simulink model "Model"  (R2023a)
settings: Solver=FixedStepAuto  StartTime=0.0  StopTime=4  FixedStep=0.0001  RelTol=1e-3
values from neighbouring files (symbols this model uses):
  J2 = 1.26e-3    (= 0.00126)    [system_init.m]
libraries: dspfdesign x4
settings Model: SimulationMode=accelerator  Creator=04  LastModifiedBy=23688
settings SolverCC: AlgebraicLoopSolver=TrustRegion
settings DataIOCC: ReturnWorkspaceOutputs=off
settings DebuggingCC: UnconnectedInputMsg=warning  UnconnectedOutputMsg=warning  UnconnectedLineMsg=warning
settings ModelReferenceCC: EnableRefExpFcnMdlSchedulingChecks=on
settings RTWCC: DLArmComputeVersion=19.05

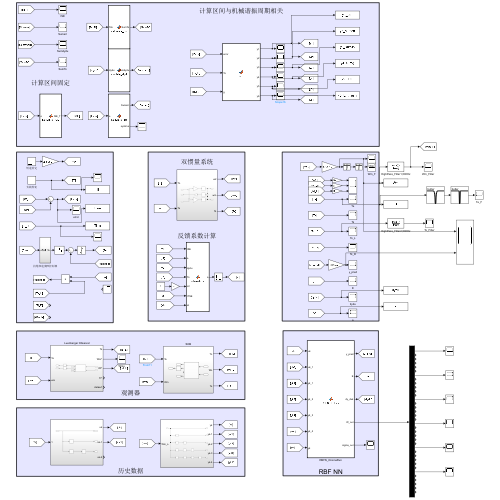
[thumbnail: Simulink's stored preview of the top-level diagram]
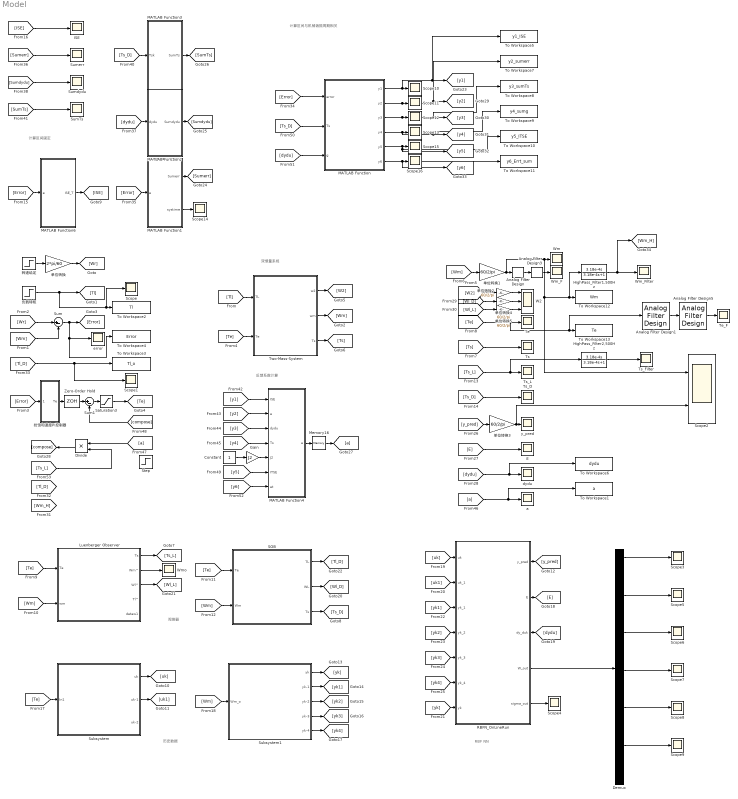
== system Model ==
  note: 观测器
  note: 历史数据
  note: 计算区间固定
  note: 计算区间与机械谐振周期相关
  note: 双惯量系统
  note: 反馈系数计算
  note: RBF NN
  " Luenberger Observer" : Subsystem
  Analog Filter Design : dspfdesign/Analog Filter Design  method=Butterworth  filttype=Bandstop  N=12  Wlo=700*2*pi  Whi=1300*2*pi  Rp=2  Rs=40
  Analog Filter Design1 : dspfdesign/Analog Filter Design  method=Butterworth  filttype=Bandstop  N=2  Wlo=700*2*pi  Whi=1300*2*pi  Rp=2  Rs=40
  Analog Filter Design3 : dspfdesign/Analog Filter Design  method=Butterworth  filttype=Bandstop  N=12  Wlo=900*2*pi  Whi=1100*2*pi  Rp=2  Rs=40
  Analog Filter Design5 : dspfdesign/Analog Filter Design  method=Butterworth  filttype=Bandstop  N=2  Wlo=950*2*pi  Whi=1050*2*pi  Rp=2  Rs=40
  Constant : Constant
  Demux : Demux  Outputs=36
  Divide : Product  Inputs=**
  E : Scope
  Gain : Gain  Gain=J2
  HighPass_Filter1,500Hz : TransferFcn  Numerator=[3.18e-4 0]  Denominator=[3.18e-4 1]
  HighPass_Filter2,500Hz : TransferFcn  Numerator=[3.18e-4 0]  Denominator=[3.18e-4 1]
  ISE : Scope
  MATLAB Function : MATLAB Function  TreatAsAtomicUnit=on
  MATLAB Function1 : MATLAB Function  TreatAsAtomicUnit=on
  MATLAB Function2 : MATLAB Function  TreatAsAtomicUnit=on
  MATLAB Function3 : MATLAB Function  TreatAsAtomicUnit=on
  MATLAB Function4 : MATLAB Function  TreatAsAtomicUnit=on
  MATLAB Function6 : MATLAB Function  TreatAsAtomicUnit=on
  Memory16 : Memory  InheritSampleTime=on
  RBFN_OnLineRun : MATLAB Function  TreatAsAtomicUnit=on
  SOB : Subsystem
  Saturation3 : Saturate  UpperLimit=2.39*3  LowerLimit=-2.39*3
  Scope{,1,3..16} (16 alike) : Scope
  Scope2 : Scope  NumInputPorts=2
  Step : Step  Time=1.2  After=0  SampleTime=0
  Subsystem : Subsystem
  Subsystem1 : Subsystem
  Sum : Sum  Inputs=|+-
  Sum1 : Sum  Inputs=|+-
  SumTs : Scope
  Sumdydu : Scope
  Sumerr : Scope
  Te : Scope
  Te_F : Scope
  To Workspace1 : ToWorkspace  VariableName=a  SampleTime=-1
  To Workspace10 : ToWorkspace  VariableName=y5_ITSE  SampleTime=-1
  To Workspace11 : ToWorkspace  VariableName=y6_Errt_sum  SampleTime=-1
  To Workspace12 : ToWorkspace  VariableName=Wm  SampleTime=-1
  To Workspace13 : ToWorkspace  VariableName=Te  SampleTime=-1
  To Workspace2 : ToWorkspace  VariableName=Tl  SampleTime=-1
  To Workspace3 : ToWorkspace  VariableName=Tl_o  SampleTime=-1
  To Workspace4 : ToWorkspace  VariableName=Error  SampleTime=-1
  To Workspace5 : ToWorkspace  VariableName=y1_ISE  SampleTime=-1
  To Workspace6 : ToWorkspace  VariableName=dydu  SampleTime=-1
  To Workspace7 : ToWorkspace  VariableName=y2_sumerr  SampleTime=-1
  To Workspace8 : ToWorkspace  VariableName=y3_sumTs  SampleTime=-1
  To Workspace9 : ToWorkspace  VariableName=y4_sumg  SampleTime=-1
  Ts : Scope
  Ts_D : Scope
  Ts_Filter : Scope
  Ts_L : Scope
  Two-Mass-System : Subsystem
  W2 : Scope  NumInputPorts=3
  Wm : Scope
  Wm_F : Scope
  Wm_Filter : Scope
  Wmo : Scope
  Zero-Order Hold : ZeroOrderHold  SampleTime=0.0005
  a : Scope
  dydu : Scope
  error : Scope
  y_pred : Scope
  单位转换 : Gain  Gain=2*pi/60
  单位转换{1..5} (5 alike) : Gain  Gain=60/2/pi
  抗饱和速度PI控制器 : Subsystem
  负载转矩 : Step  Time=0  After=0  SampleTime=0
  转速给定 : Step  Time=0.1  After=1000  SampleTime=0
  wires:
  负载转矩/1 -> Scope/1, To Workspace2/1, [Tl]
  [Tl] -> Two-Mass-System/1(TL)
  Two-Mass-System/2(wm) -> [Wm]
  [Wr] -> Sum/1
  [Wm] -> Sum/2
  Sum/1 -> To Workspace4/1, error/1, [Error]
  [Error] -> 抗饱和速度PI控制器/1(error)
  Two-Mass-System/1(w2) -> [W2]
  Two-Mass-System/3(Ts) -> [Ts]
  [Ts] -> Ts/1
  单位转换/1 -> [Wr]
  [Wm] -> 单位转换1/1
  [Te] -> " Luenberger Observer"/1(Te)
  [Wm] -> " Luenberger Observer"/2(wm)
  [Te] -> SOB/1(Te)
  [Wm] -> SOB/2(Wm)
  " Luenberger Observer"/1(Ts) -> [Ts_L]
  SOB/3(Ts) -> [Ts_D]
  [Ts_L] -> HighPass_Filter2,500Hz/1, Ts_L/1
  [Ts_D] -> Ts_D/1
  [W2] -> 单位转换2/1
  单位转换2/1 -> W2/1
  [Te] -> Subsystem/1(In1)
  Subsystem/1(uk) -> [uk]
  Subsystem/2(uk-1) -> [uk1]
  [Wm] -> Subsystem1/1(Wm_o)
  Subsystem1/1(yk) -> [yk]
  Subsystem1/2(yk-1) -> [yk1]
  Subsystem1/3(yk-2) -> [yk2]
  Subsystem1/4(yk-3) -> [yk3]
  Subsystem1/5(yk-4) -> [yk4]
  [uk] -> RBFN_OnLineRun/1(uk)
  [uk1] -> RBFN_OnLineRun/2(uk_1)
  [yk] -> RBFN_OnLineRun/7(yk)
  [yk1] -> RBFN_OnLineRun/3(yk_1)
  [yk2] -> RBFN_OnLineRun/4(yk_2)
  [yk3] -> RBFN_OnLineRun/5(yk_3)
  [yk4] -> RBFN_OnLineRun/6(yk_4)
  RBFN_OnLineRun/1(y_pred) -> [y_pred]
  RBFN_OnLineRun/2(E) -> [E]
  [E] -> E/1
  [dydu] -> To Workspace6/1, dydu/1
  [y_pred] -> 单位转换3/1
  单位转换3/1 -> Scope2/2, y_pred/1
  SOB/2(WL) -> [Wl_D]
  " Luenberger Observer"/3(Wl^) -> [Wl_L]
  单位转换4/1 -> W2/2
  [Wl_D] -> 单位转换4/1
  单位转换5/1 -> W2/3
  [Wl_L] -> 单位转换5/1
  Analog Filter Design/1 -> Analog Filter Design3/1
  Analog Filter Design3/1 -> Wm_F/1
  单位转换1/1 -> Scope2/1, HighPass_Filter1,500Hz/1, To Workspace12/1, Wm/1, Analog Filter Design/1
  [Error] -> MATLAB Function1/1(e)
  MATLAB Function1/1(Sumerr) -> [Sumerr]
  [ISE] -> ISE/1
  [Sumerr] -> Sumerr/1
  [dydu] -> MATLAB Function2/1(dydu)
  MATLAB Function2/1(Sumdydu) -> [Sumdydu]
  [Sumdydu] -> Sumdydu/1
  [Ts_D] -> MATLAB Function3/1(Tsk)
  MATLAB Function3/1(SumTs) -> [SumTs]
  [SumTs] -> SumTs/1
  [y1] -> MATLAB Function4/1(ISE)
  [y2] -> MATLAB Function4/2(e)
  [y3] -> MATLAB Function4/3(dydu)
  [y4] -> MATLAB Function4/4(Ts)
  [a] -> To Workspace1/1, a/1
  Divide/1 -> [compose]
  [Te] -> Two-Mass-System/2(Te)
  MATLAB Function6/1(ISE_T) -> [ISE]
  [Error] -> MATLAB Function6/1(e)
  Gain/1 -> MATLAB Function4/5(J2)
  Constant/1 -> Gain/1
  SOB/1(TL) -> [Tl_D]
  [Tl_D] -> To Workspace3/1, Scope1/1
  [Te] -> Analog Filter Design1/1, To Workspace13/1, Te/1
  RBFN_OnLineRun/4(W_out) -> Demux/1
  Demux/1 -> Scope3/1
  RBFN_OnLineRun/5(sigma_out) -> Scope4/1
  Demux/7 -> Scope5/1
  Demux/13 -> Scope6/1
  Demux/19 -> Scope7/1
  Demux/25 -> Scope8/1
  Demux/31 -> Scope9/1
  [compose] -> Sum1/2
  抗饱和速度PI控制器/1(Te) -> Zero-Order Hold/1
  Zero-Order Hold/1 -> Sum1/1
  [Error] -> MATLAB Function/1(error)
  MATLAB Function/1(y1) -> Scope10/1, To Workspace5/1, [y1]
  MATLAB Function/2(y2) -> Scope11/1, To Workspace7/1, [y2]
  [Ts_D] -> MATLAB Function/2(Ts)
  MATLAB Function/3(y3) -> To Workspace8/1, [y3], Scope12/1
  [dydu] -> MATLAB Function/3(g)
  MATLAB Function/4(y4) -> To Workspace9/1, [y4], Scope13/1
  MATLAB Function4/1(a) -> Memory16/1
  RBFN_OnLineRun/3(dy_duk) -> [dydu]
  Memory16/1 -> [a]
  MATLAB Function1/2(systime) -> Scope14/1
  MATLAB Function/5(y5) -> [y5], To Workspace10/1, Scope15/1
  [y5] -> MATLAB Function4/6(ITSE)
  MATLAB Function/6(y6) -> [y6], To Workspace11/1, Scope16/1
  [y6] -> MATLAB Function4/7(et)
  Analog Filter Design1/1 -> Analog Filter Design5/1
  Analog Filter Design5/1 -> Te_F/1
  HighPass_Filter2,500Hz/1 -> Ts_Filter/1
  HighPass_Filter1,500Hz/1 -> [Wm_H], Wm_Filter/1
  Sum1/1 -> Saturation3/1
  Saturation3/1 -> [Te]
  " Luenberger Observer"/2(Wm^) -> Wmo/1
  转速给定/1 -> 单位转换/1
  [Ts_L] -> Divide/2
  [a] -> Divide/1

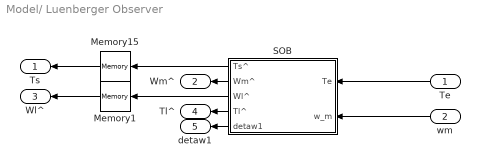
== system Model/ Luenberger Observer ==
  Te : Inport
  wm : Inport  Port=2
  Memory1 : Memory
  Memory15 : Memory
  SOB : Subsystem
  Ts : Outport
  Wm^ : Outport  Port=2
  Wl^ : Outport  Port=3
  Tl^ : Outport  Port=4
  detaw1 : Outport  Port=5
  wires:
  SOB/4(Tl^) -> Tl^/1
  SOB/1(Ts^) -> Memory15/1
  Memory15/1 -> Ts/1
  wm/1 -> SOB/2(w_m)
  SOB/2(Wm^) -> Wm^/1
  Te/1 -> SOB/1(Te)
  SOB/5(detaw1) -> detaw1/1
  Memory1/1 -> Wl^/1
  SOB/3(Wl^) -> Memory1/1

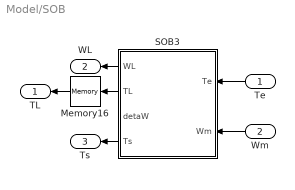
== system Model/SOB ==
  Te : Inport
  Wm : Inport  Port=2
  Memory16 : Memory
  SOB3 : Subsystem
  TL : Outport
  WL : Outport  Port=2
  Ts : Outport  Port=3
  wires:
  SOB3/1(WL) -> WL/1
  SOB3/4(Ts) -> Ts/1
  Wm/1 -> SOB3/2(Wm)
  Te/1 -> SOB3/1(Te)
  SOB3/2(TL) -> Memory16/1
  Memory16/1 -> TL/1

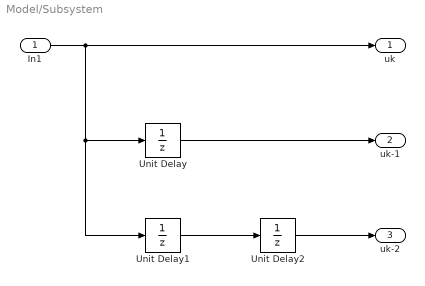
== system Model/Subsystem ==
  In1 : Inport
  Unit Delay : UnitDelay  SampleTime=-1  HasFrameUpgradeWarning=on
  Unit Delay1 : UnitDelay  SampleTime=-1  HasFrameUpgradeWarning=on
  Unit Delay2 : UnitDelay  SampleTime=-1  HasFrameUpgradeWarning=on
  uk : Outport
  uk-1 : Outport  Port=2
  uk-2 : Outport  Port=3
  wires:
  Unit Delay1/1 -> Unit Delay2/1
  Unit Delay/1 -> uk-1/1
  Unit Delay2/1 -> uk-2/1
  In1/1 -> Unit Delay1/1, Unit Delay/1, uk/1

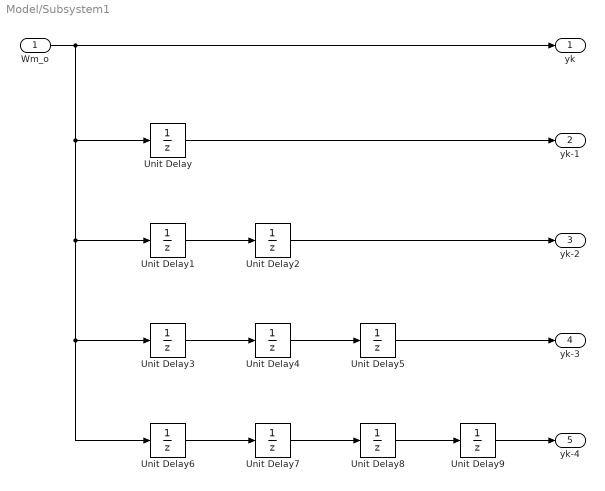
== system Model/Subsystem1 ==
  Wm_o : Inport
  Unit Delay{,1..9} (10 alike) : UnitDelay  SampleTime=-1  HasFrameUpgradeWarning=on
  yk : Outport
  yk-1 : Outport  Port=2
  yk-2 : Outport  Port=3
  yk-3 : Outport  Port=4
  yk-4 : Outport  Port=5
  wires:
  Unit Delay5/1 -> yk-3/1
  Unit Delay4/1 -> Unit Delay5/1
  Unit Delay2/1 -> yk-2/1
  Unit Delay8/1 -> Unit Delay9/1
  Unit Delay7/1 -> Unit Delay8/1
  Unit Delay6/1 -> Unit Delay7/1
  Unit Delay9/1 -> yk-4/1
  Unit Delay3/1 -> Unit Delay4/1
  Unit Delay/1 -> yk-1/1
  Wm_o/1 -> Unit Delay3/1, Unit Delay6/1, Unit Delay1/1, Unit Delay/1, yk/1
  Unit Delay1/1 -> Unit Delay2/1

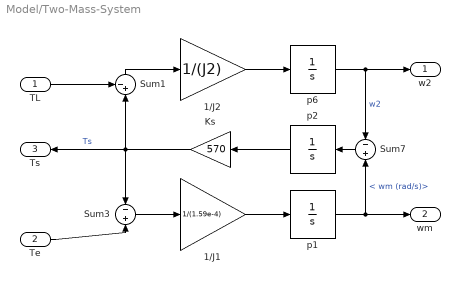
== system Model/Two-Mass-System ==
  TL : Inport
  Te : Inport  Port=2
  1/J1 : Gain  Gain=1/(1.59e-4)
  1/J2 : Gain  Gain=1/(J2)
  Ks : Gain  Gain=570
  Sum1 : Sum  Inputs=-+|
  Sum3 : Sum  Inputs=-+
  Sum7 : Sum  Inputs=-+
  p1 : TransferFcn  Denominator=[1 0]
  p2 : TransferFcn  Denominator=[1 0]
  p6 : TransferFcn  Denominator=[1 0]
  w2 : Outport
  wm : Outport  Port=2
  Ts : Outport  Port=3
  wires:
  Sum3/1 -> 1/J1/1
  1/J1/1 -> p1/1
  p1/1 -> wm/1, Sum7/2  "< wm (rad/s)>"
  p6/1 -> Sum7/1, w2/1  "w2"
  Sum7/1 -> p2/1
  Sum1/1 -> 1/J2/1
  Ks/1 -> Ts/1, Sum1/2, Sum3/1  "Ts"
  p2/1 -> Ks/1
  1/J2/1 -> p6/1
  TL/1 -> Sum1/1
  Te/1 -> Sum3/2

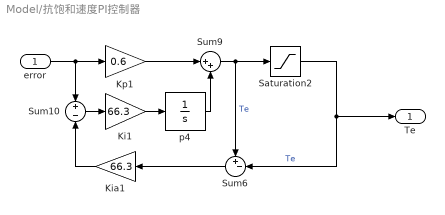
== system Model/抗饱和速度PI控制器 ==
  error : Inport
  Ki1 : Gain  Gain=66.3
  Kia1 : Gain  Gain=66.3
  Kp1 : Gain  Gain=0.6
  Saturation2 : Saturate  UpperLimit=2.39*3  LowerLimit=-2.39*3
  Sum10 : Sum  Inputs=+|-
  Sum6 : Sum  Inputs=+-|
  Sum9 : Sum  Inputs=|++
  p4 : TransferFcn  Denominator=[1 0]
  Te : Outport
  wires:
  Kia1/1 -> Sum10/2
  Sum6/1 -> Kia1/1
  Sum10/1 -> Ki1/1
  Kp1/1 -> Sum9/1
  Saturation2/1 -> Te/1, Sum6/2  "Te"
  Sum9/1 -> Sum6/1, Saturation2/1  "Te"
  p4/1 -> Sum9/2
  Ki1/1 -> p4/1
  error/1 -> Kp1/1, Sum10/1

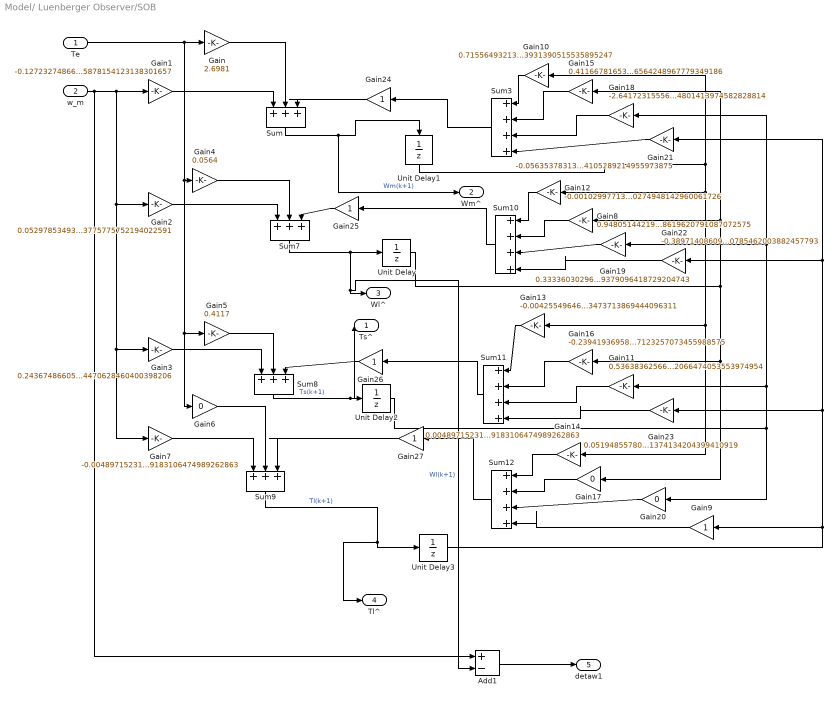
== system Model/ Luenberger Observer/SOB ==
  Te : Inport
  w_m : Inport  Port=2
  Add1 : Sum  Inputs=+-
  Gain : Gain  Gain=2.6981
  Gain1 : Gain  Gain=-0.12723274866755878154123138301657
  Gain10 : Gain  Gain=0.7155649321343931390515535895247
  Gain11 : Gain  Gain=0.53638362566622066474053553974954
  Gain12 : Gain  Gain=-0.0010299771306700274948142960061726
  Gain13 : Gain  Gain=-0.004255496467973473713869444096311
  Gain14 : Gain  Gain=0.0048971523131869183106474989262863
  Gain15 : Gain  Gain=0.41166781653316564248967779349186
  Gain16 : Gain  Gain=-0.23941936958917123257073455988575
  Gain17 : Gain  Gain=0
  Gain18 : Gain  Gain=-2.6417231555684801413974582828814
  Gain19 : Gain  Gain=0.33336030296459379096418729204743
  Gain2 : Gain  Gain=0.052978534931283775775752194022591
  Gain20 : Gain  Gain=0
  Gain21 : Gain  Gain=-0.056353783132214105289214955973875
  Gain22 : Gain  Gain=-0.38971408609680785462003882457793
  Gain23 : Gain  Gain=0.05194855780061374134204399410919
  Gain{9,24..27} (5 alike) : Gain
  Gain3 : Gain  Gain=0.24367486605714470628460400398206
  Gain4 : Gain  Gain=0.0564
  Gain5 : Gain  Gain=0.4117
  Gain6 : Gain  Gain=0
  Gain7 : Gain  Gain=-0.0048971523131869183106474989262863
  Gain8 : Gain  Gain=0.94805144219938619620791087072575
  Sum{,7..9} (4 alike) : Sum  Inputs=+++|
  Sum{3,10..12} (4 alike) : Sum  Inputs=++++|
  Unit Delay{,1..3} (4 alike) : UnitDelay  SampleTime=-1
  Ts^ : Outport
  Wm^ : Outport  Port=2
  Wl^ : Outport  Port=3
  Tl^ : Outport  Port=4
  detaw1 : Outport  Port=5
  wires:
  Te/1 -> Gain5/1, Gain6/1, Gain4/1, Gain/1
  Gain/1 -> Sum/2
  Gain1/1 -> Sum/1
  Gain4/1 -> Sum7/2
  Gain2/1 -> Sum7/1
  Gain5/1 -> Sum8/2
  Gain3/1 -> Sum8/1
  Gain6/1 -> Sum9/2
  Gain7/1 -> Sum9/1
  Sum/1 -> Unit Delay1/1, Wm^/1  "Wm(k+1)"
  Sum7/1 -> Add1/2, Wl^/1, Unit Delay/1  "Wl(k+1)"
  Sum8/1 -> Ts^/1, Unit Delay2/1  "Ts(k+1)"
  Sum9/1 -> Tl^/1, Unit Delay3/1  "Tl(k+1)"
  Sum12/1 -> Gain27/1
  Gain10/1 -> Sum3/1
  Gain11/1 -> Sum11/3
  Gain9/1 -> Sum12/4
  Gain12/1 -> Sum10/1
  Gain13/1 -> Sum11/1
  Gain14/1 -> Sum12/1
  Gain17/1 -> Sum12/2
  Gain19/1 -> Sum10/3
  Unit Delay1/1 -> Gain14/1, Gain13/1, Gain12/1, Gain10/1
  Unit Delay/1 -> Gain8/1, Gain15/1, Gain17/1, Gain16/1
  Unit Delay2/1 -> Gain11/1, Gain18/1, Gain19/1, Gain20/1
  Unit Delay3/1 -> Gain21/1, Gain22/1, Gain23/1, Gain9/1
  Gain25/1 -> Sum7/3
  Gain26/1 -> Sum8/3
  Sum3/1 -> Gain24/1
  Gain24/1 -> Sum/3
  Gain15/1 -> Sum3/2
  Gain18/1 -> Sum3/3
  Gain21/1 -> Sum3/4
  Sum10/1 -> Gain25/1
  Gain8/1 -> Sum10/2
  Sum11/1 -> Gain26/1
  Gain16/1 -> Sum11/2
  Gain23/1 -> Sum11/4
  Gain27/1 -> Sum9/3
  Gain20/1 -> Sum12/3
  Gain22/1 -> Sum10/4
  Add1/1 -> detaw1/1
  w_m/1 -> Add1/1, Gain3/1, Gain7/1, Gain2/1, Gain1/1

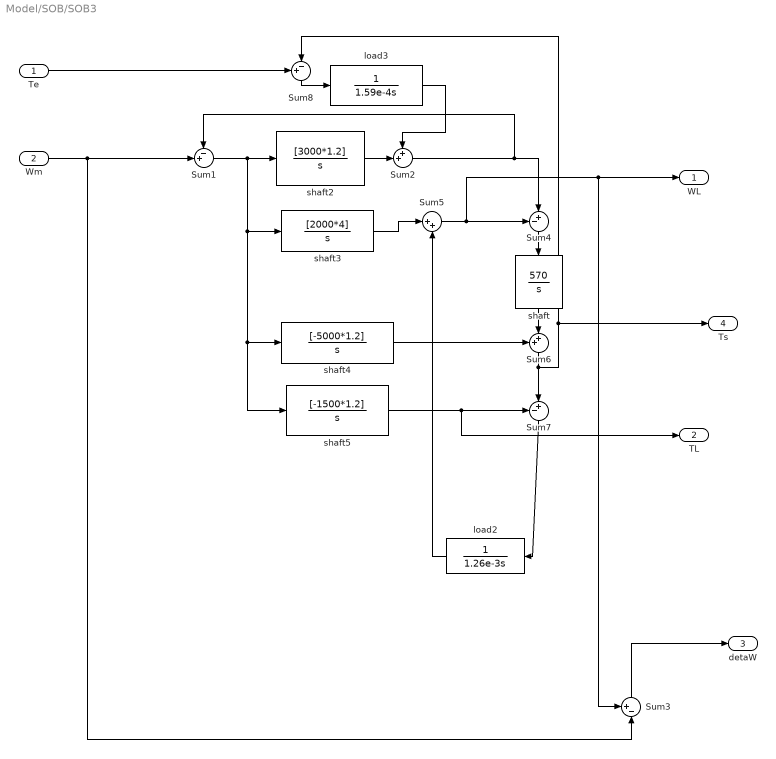
== system Model/SOB/SOB3 ==
  Te : Inport
  Wm : Inport  Port=2
  Sum1 : Sum  Inputs=-+|
  Sum2 : Sum  Inputs=++|
  Sum3 : Sum  Inputs=+-|
  Sum4 : Sum  Inputs=-+|
  Sum5 : Sum  Inputs=|++
  Sum6 : Sum  Inputs=++|
  Sum7 : Sum  Inputs=-+|
  Sum8 : Sum  Inputs=+-|
  load2 : TransferFcn  Denominator=[1.26e-3 0]
  load3 : TransferFcn  Denominator=[1.59e-4 0]
  shaft : TransferFcn  Numerator=[570]  Denominator=[1 0]
  shaft2 : TransferFcn  Numerator=[3000*1.2]  Denominator=[1 0]
  shaft3 : TransferFcn  Numerator=[2000*4]  Denominator=[1 0]
  shaft4 : TransferFcn  Numerator=[-5000*1.2]  Denominator=[1 0]
  shaft5 : TransferFcn  Numerator=[-1500*1.2]  Denominator=[1 0]
  WL : Outport  VectorParamsAs1DForOutWhenUnconnected=off
  TL : Outport  Port=2  VectorParamsAs1DForOutWhenUnconnected=off
  detaW : Outport  Port=3  VectorParamsAs1DForOutWhenUnconnected=off
  Ts : Outport  Port=4  VectorParamsAs1DForOutWhenUnconnected=off
  wires:
  Wm/1 -> Sum1/2, Sum3/2
  Te/1 -> Sum8/1
  load3/1 -> Sum2/1
  Sum8/1 -> load3/1
  load2/1 -> Sum5/2
  Sum7/1 -> load2/1
  Sum6/1 -> Sum7/2, Ts/1, Sum8/2
  shaft5/1 -> TL/1, Sum7/1
  shaft/1 -> Sum6/2
  shaft4/1 -> Sum6/1
  Sum4/1 -> shaft/1
  Sum5/1 -> WL/1, Sum3/1, Sum4/1
  shaft3/1 -> Sum5/1
  Sum2/1 -> Sum4/2, Sum1/1
  shaft2/1 -> Sum2/2
  Sum1/1 -> shaft5/1, shaft4/1, shaft3/1, shaft2/1
  Sum3/1 -> detaW/1

== matlab function Model/RBFN_OnLineRun ==
  settings: updateMethod=DISCRETE  sampleTime=0.0001
  data: y_pred output; uk input; E output; uk_1 input; yk_1 input; yk_2 input; yk_3 input; yk_4 input; yk input; dy_duk output; W_out output; sigma_out output
function [y_pred, E, dy_duk, W_out, sigma_out]  = RBFN_OnLine(uk, uk_1, yk_1, yk_2, yk_3, yk_4, yk)

%6个输入，包含当前、过去输入与过去输出
u = [uk; uk_1; yk_1; yk_2; yk_3; yk_4]; % [6 x 1]

%RBFN参数定义与初始化
persistent centers sigma W learning

if isempty(centers)
    %从文件中加载预训练的参数，注意文件名
    data = load('RBFN_parameters2.mat');
    centers = data.centers;
    sigma = data.sigma;
    W = data.W_init;
    learning = true;
end

K = 36; % 神经元数量
H = zeros(K, 1);

% 计算偏导数
delta = zeros(K, 1); 

for j = 1:K
    % 计算第 j 个 RBF 神经元的输出
    distance = norm(u - centers(j, :)'); 
    H(j) = exp(- (distance^2) / (2 * sigma^2));

    % c_{j1} 是 centers 矩阵的第 j 行，第1个元素，也就是uk所具体对应的中心值，因为有36个神经元，所以对应36个值
    delta(j) = uk - centers(j, 1);
end

% 计算网络的预测输出
y_pred = W' * H;

% 计算预测误差
e = yk - y_pred;
E = e;

% 学习率设置
eta_W = 0.10;    
eta_c = 0.008;    
eta_sigma = 0.005; 

epsilon = 0.01; % 误差阈值

% 判断是否需要更新参数，误差没有达到要求就更新
if learning
    W = W + eta_W * e * H;

    for j = 1:K
        centers(j, :) = centers(j, :) + ...
            eta_c * e * W(j) * H(j) * (u' - centers(j, :)) / sigma^2;
    end

    delta_sigma = 0;

    for j = 1:K
        delta_sigma = delta_sigma + ...
            e * W(j) * H(j) * (norm(u - centers(j, :)')^2) / sigma^3;
    end
    
    sigma = sigma + eta_sigma * delta_sigma / K;
end

% 收敛条件判断
if abs(e) < epsilon
    % 误差小于阈值，停止参数更新
    learning = false;
else
    % 误差大于阈值，继续参数更新
    learning = true;
end

% 计算网络输出 y 关于当前输入 u_k 的偏导数

% 推导公式：
% dy/du_k = -(1 / sigma^2) * sum_{j=1}^K [ W_j * H_j * (u_k - c_{j1})]

% 计算偏导数，计算结果是当前时刻
dy_duk = - (1 / sigma^2) * sum(W .* H .* delta);
W_out = W;
sigma_out = sigma;

end

== matlab function Model/MATLAB Function ==
  settings: updateMethod=DISCRETE
  data: error input; y1 output; y2 output; Ts input; y3 output; g input; y4 output; y5 output; y6 output
function [y1, y2, y3, y4, y5, y6]  = fcn(error, Ts, g)

persistent T time err_last err_squa err_sum err_squa_t ISE_output Err_output ISE_New ISE_Old Err_New Err_Old Ts_sum Ts_output Ts_New Ts_Old g_sum g_New g_Old g_output ITSE_New ITSE_Old ITSE_output Errt_New Errt_Old Errt_sum Errt_output
if isempty(T)
    T = 0.0001;                                        % 系统运行周期，s
    time = 0;                                          % 系统运行计时

    err_last = 0;                                      % 上一时刻误差
    err_squa = 0;                                      % 误差平方
    err_squa_t = 0;                                    % 误差平方时间加权
    err_sum = 0;                                       % 误差求和

    ISE_output = 0;                                    % ISE计算输出
    ITSE_output = 0;                                   % ITSE输出
    Err_output = 0;                                    % 误差求和输出

    ISE_New = 0;                                       % ISE新值
    ISE_Old = 0;                                       % ISE旧值

    Err_New = 0;                                       % 误差和新值
    Err_Old = 0;                                       % 误差和旧值

    Ts_sum = 0;                                        % 扭矩求和
    Ts_Old = 0;                                        % 求和旧值
    Ts_New = 0;                                        % 求和新值
    Ts_output = 0;                                     % 扭矩求和输出

    g_sum = 0;                                         % 梯度求和
    g_New = 0;                                         % 求和新值
    g_Old = 0;                                         % 求和旧值
    g_output = 0;                                      % 梯度求和输出

    ITSE_New = 0;                                      % ITSE新值
    ITSE_Old = 0;                                      % ITSE旧值

    Errt_New = 0;                                      % 误差时间加权新值
    Errt_Old = 0;                                      % 误差时间加权旧值
    Errt_output = 0;                                   % 误差时间加权输出
    Errt_sum = 0;                                      % 误差时间加权

end

if (time > 0.242)  % 运行进入稳态再计算
    if (sign(error) == sign(err_last))  % 未过零，累加需要的变量

        err_squa = err_squa + (error^2);
        err_squa_t = err_squa_t + ((error^2) * time);  % 使用时间项
        err_sum = error + err_sum;
        Errt_sum = (error * time) + Errt_sum;
        Ts_sum = Ts + Ts_sum;
        
        if(abs(error) > 0.01)
            g_sum = g + g_sum;
        else
            g_sum = g_sum;
        end

    else                                % 过零，输出上半周期结果

        ISE_New = err_squa * T;
        ITSE_New = (err_squa_t * T);
        Err_New = err_sum;
        Errt_New = Errt_sum;
        Ts_New = Ts_sum;
        g_New = g_sum;

        ISE_output = ISE_New * 0.68 + ISE_Old * 0.32;
        ITSE_output = ITSE_New * 0.74 + ITSE_Old * 0.26;
        Err_output = Err_New * 0.8 + Err_Old * 0.2;
        Errt_output = Errt_New * 0.7 + Errt_Old * 0.3;
        Ts_output = Ts_New * 0.68 + Ts_Old * 0.32;
        g_output = g_New * 0.8 + g_Old * 0.2;

        err_squa = 0;
        err_squa_t = 0;
        err_sum = 0;
        Errt_sum = 0;
        Ts_sum = 0;

        if(abs(error) > 0.01)
            g_sum = 0;
        else
            g_sum = g_sum;
        end

    end
end

% 数据传递
time = time + T;
err_last = error;

ISE_Old = ISE_output;
ITSE_Old = ITSE_output;
Err_Old = Err_output;
Errt_Old = Errt_output;
Ts_Old = Ts_output;
g_Old = g_output;

% 小数位控制
ISE_output = round(ISE_output*1000)/1000;
ITSE_output = round(ITSE_output*1000)/1000;
Err_output = round(Err_output*1000)/1000;
Errt_output = round(Errt_output*1000)/1000;
Ts_output = round(Ts_output*1000)/1000;
g_output = round(g_output*1000)/1000; 

% 结果输出
y1 = ISE_output;                                       % 半个谐振周期ISE
y2 = Err_output;                                       % 半个谐振周期误差和
y3 = Ts_output;                                        % 半个谐振周期扭矩和
y4 = g_output;                                         % 半个谐振周期梯度和
y5 = ITSE_output;                                      % 半个谐振周期ITSE
y6 = Errt_output;                                      % 半个谐振周期时间加权误差和

== matlab function Model/MATLAB Function1 ==
  settings: updateMethod=DISCRETE  sampleTime=0.0001
  data: e input; Sumerr output; systime output
function [Sumerr, systime] = calculate_err(e)

persistent T time Err M ErrOut Err_1

if isempty(T)
    T = 0.0001;
    time = 0;
    Err = 0;
    M = 0;
    ErrOut = 0;
    Err_1 = 0;
end

if (time > 1)

    Err = Err_1 + e;
    M = M + 1;
    Err_1 = Err;

    if (M == 10)
        ErrOut = Err*0.9 + ErrOut*0.1;
        Err = 0;
        Err_1 = 0;
        M = 0;
    end

end

time = time + T;

Sumerr = round(ErrOut*1000)/1000;
systime = time;

end

== matlab function Model/MATLAB Function2 ==
  settings: updateMethod=DISCRETE  sampleTime=0.0001
  data: dydu input; Sumdydu output
function Sumdydu = calculate_dydu(dydu)

persistent T time dydu_sum M dyduOut

if isempty(T)
    T = 0.0001;
    time = 0;
    dydu_sum = 0;
    M = 0;
    dyduOut = 0;
end

if (time > 1)

    dydu_sum = dydu_sum + dydu;
    M = M + 1;

    if (M == 10)
        % 低通滤波，取70%当前值和30%的历史值
        dyduOut = dyduOut*0.3 + dydu_sum*0.7;
        dydu_sum = 0;
        M = 0;
    end

end

time = time + T;

Sumdydu = round(dyduOut*1000)/1000;

end

== matlab function Model/MATLAB Function3 ==
  settings: updateMethod=DISCRETE  sampleTime=0.0001
  data: Tsk input; SumTs output
function SumTs = calculate_Ts(Tsk)

persistent T time Ts_sum M TsOut

if isempty(T)
    T = 0.0001;
    time = 0;
    Ts_sum = 0;
    M = 0;
    TsOut = 0;
end

if (time > 1)

    Ts_sum = Ts_sum + Tsk;
    M = M + 1;

    if (M == 10)
        % 低通滤波，取70%当前值和30%的历史值
        TsOut = TsOut*0.3 + Ts_sum*0.7;
        Ts_sum = 0;
        M = 0;
    end

end

time = time + T;

SumTs = round(TsOut*1000)/1000;

end

== matlab function Model/MATLAB Function4 ==
  settings: updateMethod=DISCRETE
  data: ISE input; a output; e input; dydu input; Ts input; J2 input; ITSE input; et input
function a = calculate_a(ISE,e,dydu,Ts,J2,ITSE,et)
persistent T time a_now a_old eta_a1 eta_a2 cnt

if isempty(T)
    T = 0.0001;
    time = 0;
    a_old = 0.0;
    a_now = 0.0;
    cnt = 0;
    % eta_a1 = 0.500;   % 评价函数为ISE+ITSE的学习率，要小一点
    eta_a1 = 0.740;     % 评价函数为ITSE的学习率，要大一点
    % eta_a2 = 0.500;   % 评价函数为ISE+ITSE的学习率，要小一点
    eta_a2 = 0.740;     % 评价函数为ITSE的学习率，要大一点
end

if (time >= 1.2 && cnt > 50)
    if (ISE > 0.005)
        if(J2 == 1.26e-3)
            % a_now = a_old - eta_a1 * ((2 * ISE * e * dydu * Ts) + (2 * ITSE * et * dydu * Ts));     % 评价函数为ISE+ITSE
            a_now = a_old - eta_a1 * ((2 * ITSE * et * dydu * Ts));                                   % 评价函数为ITSE
            if (a_now > 1.4)
                a_now = 1.4;
            end

            if (a_now < 0)
                a_now = abs(a_now);
                if (a_now >1.4)
                    a_now = 1.4;
                end
            end
        end
        if(J2 == 4.35e-3)
            % a_now = a_old - eta_a2 * ((2 * ISE * e * dydu * Ts) + (2 * ITSE * et * dydu * Ts));   % 评价函数为ISE+ITSE
            a_now = a_old - eta_a2 * ((2 * ITSE * et * dydu * Ts));                                 % 评价函数为ITSE
            if (a_now > 1.4)
                a_now = 1.4;
            end

            if (a_now < 0)
                a_now = abs(a_now);
                if (a_now >1.4)
                    a_now = 1.4;
                end
            end
        end
    else
        a_now = a_old;
    end
    cnt = 0;
end

time = time + T;
cnt = cnt + 1;

a = a_now;
a_old = a_now;

end

== matlab function Model/MATLAB Function6 ==
  settings: updateMethod=DISCRETE  sampleTime=0.0001
  data: e input; ISE_T output
function ISE_T = calculate_ISE(e)

persistent T time M SumErr SumISE

if isempty(T)
    T = 0.0001;
    time = 0;
    SumErr = 0;
    SumISE = 0;
    M = 0;
end

if (time >= 1)

    SumErr = SumErr + e^2 * T;
    M = M + 1;
    
    % 计算周期为0.01，100个仿真步长
    if (M == 100)
        % 低通滤波，取70%当前值和30%的历史值
        SumISE = SumErr*0.7 + SumISE*0.3;
        SumErr = 0;
        M = 0;
    end

end

time = time + T;

% 最终结果保留三位小数，保留小数的操作主要是为了不要让数值抖动太大
ISE_T = round(SumISE*1000)/1000;

end
